simulink model "simulation_model"  (R2023a)
settings: Solver=ode4  StartTime=0.0  StopTime=end_time  FixedStep=dt  MaxStep=0.001  RelTol=1e-3
values from neighbouring files (symbols this model uses):
  dt = 0.001    [sim_test_script.m]
  IC = [x_ic, theta_ic, D_x_ic, D_theta_ic]'    [sim_test_script.m]
settings Model: Creator=Adam  LastModifiedBy=Adam
settings SolverCC: AlgebraicLoopSolver=TrustRegion
settings DataIOCC: SaveOutput=off  SignalLogging=off  DSMLogging=off
settings DebuggingCC: AlgebraicLoopMsg=none  UnconnectedInputMsg=warning  UnconnectedOutputMsg=warning  UnconnectedLineMsg=warning
settings ModelReferenceCC: EnableRefExpFcnMdlSchedulingChecks=on
settings RTWCC: DLArmComputeVersion=19.05

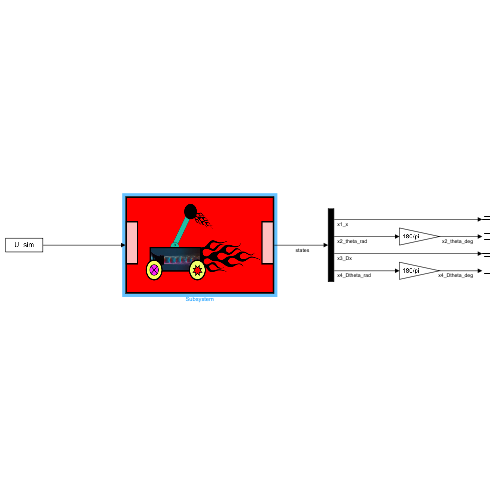
[thumbnail: Simulink's stored preview of the top-level diagram]
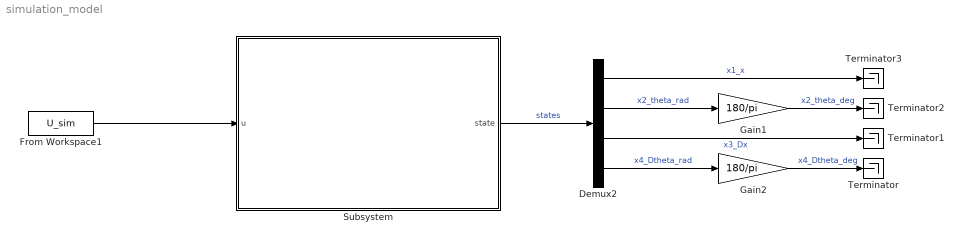
== system simulation_model ==
  Demux2 : Demux
  From Workspace1 : FromWorkspace  VariableName=U_sim  SampleTime=dt
  Gain1 : Gain  Gain=180/pi
  Gain2 : Gain  Gain=180/pi
  Subsystem : Subsystem
      mask Display: image('D:\zpy_projects\wahadlo\images_drawio\wahadlo-wahadlo_alone_mk2.png'); % Use "Edit Image" on toolstrip to change.
  Terminator{,1..3} (4 alike) : Terminator
  wires:
  Gain2/1 -> Terminator/1  "x4_Dtheta_deg"
  Demux2/4 -> Gain2/1  "x4_Dtheta_rad"
  Demux2/3 -> Terminator1/1  "x3_Dx"
  Demux2/2 -> Gain1/1  "x2_theta_rad"
  Demux2/1 -> Terminator3/1  "x1_x"
  Gain1/1 -> Terminator2/1  "x2_theta_deg"
  Subsystem/1(state) -> Demux2/1  "states"
  From Workspace1/1 -> Subsystem/1(u)

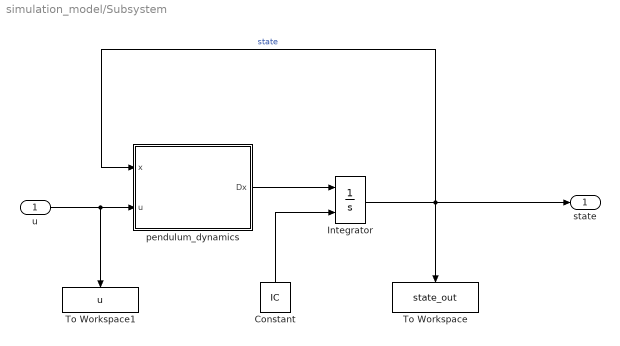
== system simulation_model/Subsystem ==
  u : Inport
  Constant : Constant  Value=IC
  Integrator : Integrator  InitialConditionSource=external
  To Workspace : ToWorkspace  VariableName=state_out  SampleTime=-1
      settings: Save2DSignal=2-D array (concatenate along first dimension)
  To Workspace1 : ToWorkspace  VariableName=u  SampleTime=-1
  pendulum_dynamics : MATLAB Function  TreatAsAtomicUnit=on
  state : Outport
  wires:
  Integrator/1 -> state/1, pendulum_dynamics/1(x), To Workspace/1  "state"
  u/1 -> pendulum_dynamics/2(u), To Workspace1/1
  pendulum_dynamics/1(Dx) -> Integrator/1
  Constant/1 -> Integrator/2

== matlab function simulation_model/Subsystem/pendulum_dynamics ==
  data: x input; u input; Dx output; params parameter
function Dx = dynamika_wahadla(x, u, params)
% x : state
% u : input signal
%
% params scope: "parameters"

% State, function input: x = [x Dx theta Dtheta]'
x1 = x(1);
x2 = x(2);
x3 = x(3);
x4 = x(4);

% % Sat na x1   
% if x1 >= 0.4
%     x1 = 0.4;
% elseif x1 <= -0.4
%     x1 = -0.4;
% end

% Params
params = num2cell(params);
[M, mc, mp, Lp, Lc, g, b, gamma, D, alpha, mr, Mt, L, Jcm, Jt] = params{:};
% M       = params(1);
% mc      = params(2);
% mp      = params(3);
% Lp      = params(4);
% Lc      = params(5);
% g       = params(6);
% b       = params(7);
% gamma   = params(8);
% D       = params(9);
% alpha   = params(10);
% mr      = params(11);
% Mt      = params(12);
% L       = params(13);
% Jcm     = params(14);
% Jt      = params(15);

% Equations for pendulum dynamics
den = Jt*Mt - L^2 * mr^2 * cos(x2);
ddt_x1 = x3;
ddt_x2 = x4;
ddt_x3 = ( Jt*(D*cos(alpha) + ...
           L*mr*x4^2*sin(x2) - ...
           b*x3 + u) - ...
           L*mr*cos(x2) * ( D*( L*cos(alpha-x2) + sin(alpha+pi/4) ) + ...
           L*g*mr*sin(x2) - gamma*x4 ) ) / den;

ddt_x4 = ( -L*mr*cos(x2) * (D*cos(alpha) + ...
           L*mr*x4^2*sin(x2) - ...
           b*x3 + u) + ...
           Mt * ( D*( L*cos(alpha-x2) + sin(alpha+pi/4) ) + ... 
           L*g*mr*sin(x2) - ... 
           gamma*x4 ) ) / den;

% output
Dx = [ddt_x1 ddt_x2 ddt_x3 ddt_x4]';

end
